simulink model "Open_Loop_Question_A"  (R2016a)
settings: Solver=ode45  StartTime=0.0  StopTime=10.0  RelTol=1e-3
values from neighbouring files (symbols this model uses):
  A = [0,1,0,0;20.9,0,0,0;0,0,0,1;-0.8,0,0,0]    [SSAE_script.m]
  B = [0;-1;0;0.5]    [SSAE_script.m]
  C = [1,0,0,0;0,0,1,0]    [SSAE_script.m]
settings Model: Creator=el12074  LastModifiedBy=dimst
settings DataIOCC: LimitDataPoints=on  SaveFormat=Array
settings DebuggingCC: SolverPrmCheckMsg=warning
settings HardwareCC: ProdBitPerPointer=32  ProdLargestAtomicFloat=None  ProdIntDivRoundTo=Undefined  ProdEndianess=Unspecified  ProdWordSize=32  ProdHWDeviceType=32-bit Generic
settings ModelReferenceCC: PropagateSignalLabelsOutOfModel=off
settings ConfigComp: CovModelRefEnable=Off  CovSFcnEnable=off

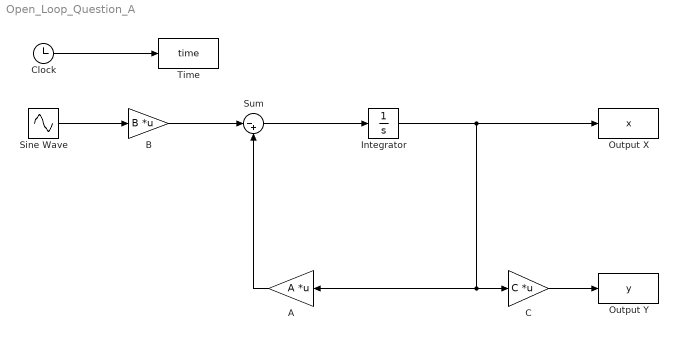
== system Open_Loop_Question_A ==
  A : Gain  Gain=A  Multiplication=Matrix(K*u)
  B : Gain  Gain=B  Multiplication=Matrix(K*u)
  C : Gain  Gain=C  Multiplication=Matrix(K*u)
  Clock : Clock
  Integrator : Integrator
  Output X : ToWorkspace  VariableName=x  SaveFormat=Timeseries  SampleTime=-1
  Output Y : ToWorkspace  VariableName=y  SaveFormat=Timeseries  SampleTime=-1
  Sine Wave : Sin  SampleTime=0
  Sum : Sum  Inputs=|-+
  Time : ToWorkspace  VariableName=time  SaveFormat=Timeseries  SampleTime=-1
  wires:
  Sine Wave/1 -> B/1
  B/1 -> Sum/1
  A/1 -> Sum/2
  Sum/1 -> Integrator/1
  Integrator/1 -> Output X/1, C/1, A/1
  C/1 -> Output Y/1
  Clock/1 -> Time/1
